simulink model "harness_plant_attitude_test"  (R2025a)
settings: Solver=VariableStepAuto  StartTime=0.0  StopTime=10.0  RelTol=1e-3
settings Model: Creator=Jackt  LastModifiedBy=Jackt

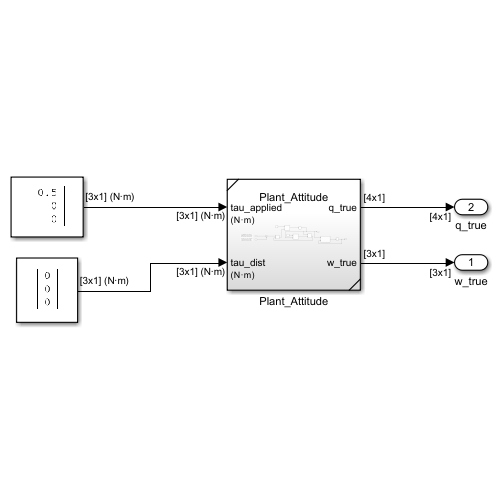
[thumbnail: Simulink's stored preview of the top-level diagram]
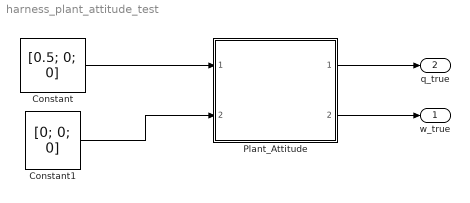
== system harness_plant_attitude_test ==
  Constant : Constant  Value=[0.5; 0; 0]  VectorParams1D=off
  Constant1 : Constant  Value=[0; 0; 0]  VectorParams1D=off
  Plant_Attitude : Subsystem  ReferencedSubsystem=Plant_Attitude
  w_true : Outport
  q_true : Outport  Port=2
  wires:
  Constant/1 -> Plant_Attitude/1
  Constant1/1 -> Plant_Attitude/2
  Plant_Attitude/2 -> w_true/1
  Plant_Attitude/1 -> q_true/1
